simulink model "loan"  (R2024b)
settings: Solver=VariableStepAuto  StartTime=0.0  StopTime=70  RelTol=1e-3
settings Model: Creator=Botló  LastModifiedBy=Botló

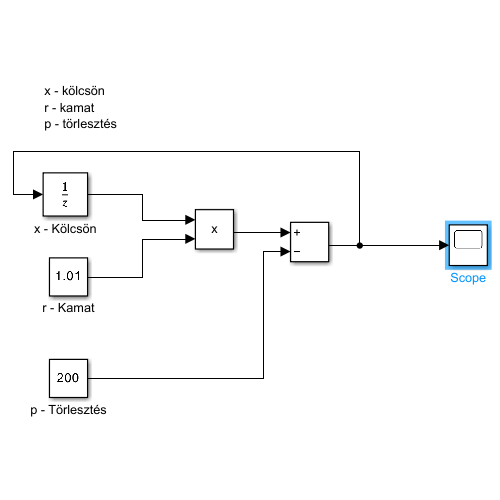
[thumbnail: Simulink's stored preview of the top-level diagram]
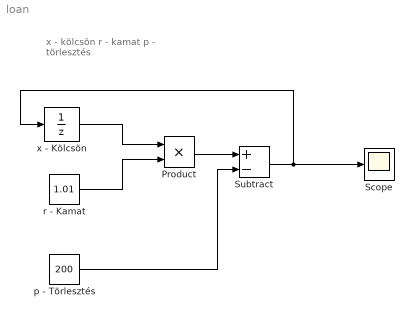
== system loan ==
  note: x - kölcsön
      | r - kamat
      | p - törlesztés
  Product : Product
  Scope : Scope
  Subtract : Sum  Inputs=+-
  p - Törlesztés : Constant  Value=200
  r - Kamat : Constant  Value=1.01
  x - Kölcsön : UnitDelay  InitialCondition=10000  HasFrameUpgradeWarning=on
  wires:
  x - Kölcsön/1 -> Product/1
  r - Kamat/1 -> Product/2
  Product/1 -> Subtract/1
  p - Törlesztés/1 -> Subtract/2
  Subtract/1 -> Scope/1, x - Kölcsön/1
